simulink model "LAB7"  (R2025b)
settings: Solver=VariableStepAuto  StartTime=0.0  StopTime=100  RelTol=1e-3
settings Model: Creator=Wingshingsho  LastModifiedBy=Wingshingsho

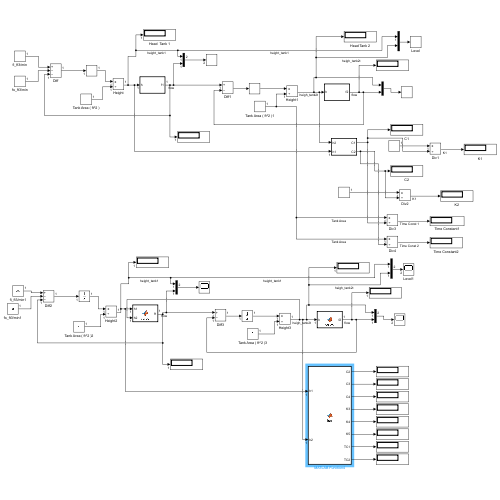
[thumbnail: Simulink's stored preview of the top-level diagram]
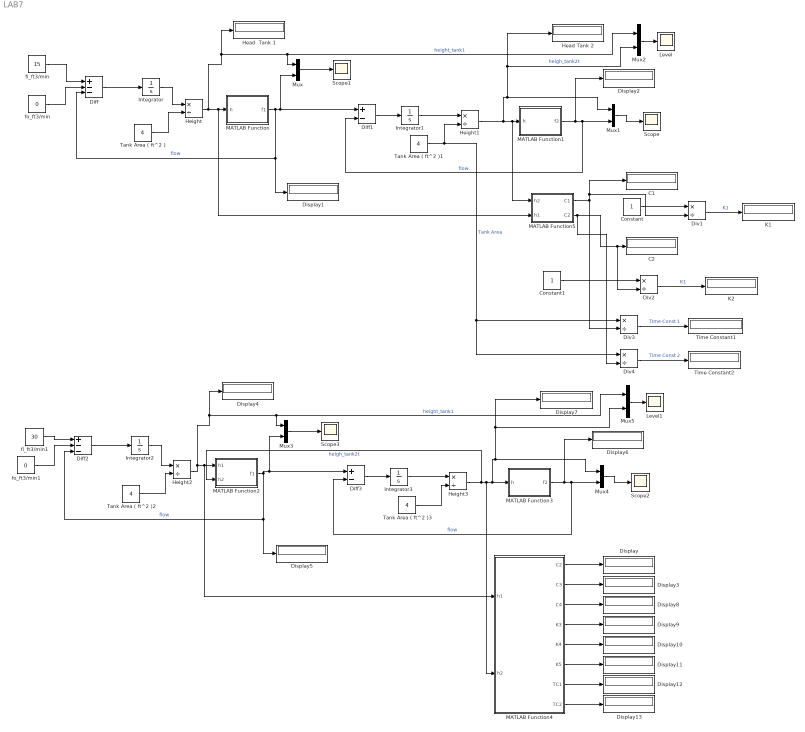
== system LAB7 ==
  C1 : Display
  C2 : Display
  Constant : Constant
  Constant1 : Constant
  Diff : Sum  Inputs=+--
  Diff1 : Sum  Inputs=+-
  Diff2 : Sum  Inputs=+--
  Diff3 : Sum  Inputs=+-
  Display{,1..13} (14 alike) : Display
  Div{1..4} (4 alike) : Product  Inputs=*/
  Head  Tank 1 : Display
  Head Tank 2 : Display
  Height{,1..3} (4 alike) : Product  Inputs=*/
  Integrator{,1..3} (4 alike) : Integrator
  K1 : Display
  K2 : Display
  Level : Scope
      settings: ActiveDisplayYMinimum=-1  ActiveDisplayYMaximum=1  DataLoggingVariableName=ScopeData2
  Level1 : Scope
      settings: ActiveDisplayYMinimum=-5.1866326305686812  ActiveDisplayYMaximum=46.679693675118138  DataLoggingVariableName=ScopeData3
  MATLAB Function : MATLAB Function  TreatAsAtomicUnit=on
  MATLAB Function1 : MATLAB Function  TreatAsAtomicUnit=on
  MATLAB Function2 : MATLAB Function  TreatAsAtomicUnit=on
  MATLAB Function3 : MATLAB Function  TreatAsAtomicUnit=on
  MATLAB Function4 : MATLAB Function  TreatAsAtomicUnit=on
  MATLAB Function5 : MATLAB Function  TreatAsAtomicUnit=on
  Mux{,1..5} (6 alike) : Mux  Inputs=2
  Scope{,1..3} (4 alike) : Scope
      Scope settings: ActiveDisplayYMinimum=-1  ActiveDisplayYMaximum=1
      Scope1 settings: ActiveDisplayYMinimum=-1  ActiveDisplayYMaximum=1
      Scope2 settings: ActiveDisplayYMinimum=-1  ActiveDisplayYMaximum=1  DataLoggingVariableName=ScopeData4
      Scope3 settings: ActiveDisplayYMinimum=-3.7438754161647805  ActiveDisplayYMaximum=33.694878745483031  DataLoggingVariableName=ScopeData5
  Tank Area ( ft^2 ){,1..3} (4 alike) : Constant  Value=4
  Time Constant1 : Display
  Time Constant2 : Display
  fi_ft3/min : Constant  Value=15
  fi_ft3/min1 : Constant  Value=30
  fo_ft3/min : Constant  Value=0
  fo_ft3/min1 : Constant  Value=0
  wires:
  fi_ft3/min/1 -> Diff/1
  fo_ft3/min/1 -> Diff/2
  Diff/1 -> Integrator/1
  Integrator/1 -> Height/1
  Tank Area ( ft^2 )/1 -> Height/2
  Height/1 -> Head  Tank 1/1, Mux2/1, Mux/1, MATLAB Function5/2(h1), MATLAB Function/1(h)  "height_tank1"
  MATLAB Function/1(f1) -> Diff/3, Display1/1, Diff1/1, Mux/2  "flow"
  Diff1/1 -> Integrator1/1
  Integrator1/1 -> Height1/1
  Tank Area ( ft^2 )1/1 -> Div4/1, Div3/1, Height1/2  "Tank Area"
  Height1/1 -> Mux2/2, Head Tank 2/1, Mux1/1, MATLAB Function5/1(h2), MATLAB Function1/1(h)  "heigh_tank2t"
  MATLAB Function1/1(f2) -> Display2/1, Mux1/2, Diff1/2  "flow"
  Mux/1 -> Scope1/1
  Mux1/1 -> Scope/1
  Mux2/1 -> Level/1
  Mux4/1 -> Scope2/1
  Height3/1 -> MATLAB Function2/2(h2), MATLAB Function4/2(h2), Mux5/2, Display7/1, Mux4/1, MATLAB Function3/1(h)  "heigh_tank2t"
  Mux3/1 -> Scope3/1
  MATLAB Function3/1(f2) -> Display6/1, Mux4/2, Diff3/2  "flow"
  Tank Area ( ft^2 )3/1 -> Height3/2
  Mux5/1 -> Level1/1
  MATLAB Function2/1(f1) -> Diff3/1, Mux3/2, Diff2/3, Display5/1  "flow"
  Height2/1 -> Display4/1, Mux5/1, Mux3/1, MATLAB Function4/1(h1), MATLAB Function2/1(h1)  "height_tank1"
  Integrator3/1 -> Height3/1
  Diff3/1 -> Integrator3/1
  Diff2/1 -> Integrator2/1
  fo_ft3/min1/1 -> Diff2/2
  fi_ft3/min1/1 -> Diff2/1
  Integrator2/1 -> Height2/1
  Tank Area ( ft^2 )2/1 -> Height2/2
  MATLAB Function5/1(C1) -> Div1/2, C1/1, Div3/2
  MATLAB Function5/2(C2) -> Div4/2, Div2/2, C2/1
  Constant/1 -> Div1/1
  Div1/1 -> K1/1  "K1"
  Constant1/1 -> Div2/1
  Div2/1 -> K2/1  "K1"
  Div3/1 -> Time Constant1/1  "TIme Const 1"
  Div4/1 -> Time Constant2/1  "Time Const 2"
  MATLAB Function4/1(C2) -> Display/1
  MATLAB Function4/2(C3) -> Display3/1
  MATLAB Function4/3(C4) -> Display8/1
  MATLAB Function4/4(K3) -> Display9/1
  MATLAB Function4/5(K4) -> Display10/1
  MATLAB Function4/6(K5) -> Display11/1
  MATLAB Function4/7(TC1) -> Display12/1
  MATLAB Function4/8(TC2) -> Display13/1

== matlab function LAB7/MATLAB Function1 ==
  data: h input; f2 output
function f2 = valve(h)
Cv = 75 * 0.13336;
LHO = 70;
SG = LHO / 62.4;
Pressure = ( LHO * h )/144;
f2 = Cv * (SG)^-0.5 * ((Pressure)^0.5);

end

== matlab function LAB7/MATLAB Function ==
  data: h input; f1 output
function f1 = valve(h)
Cv = 75 * 0.13336;
LHO = 70;
SG = LHO / 62.4;
Pressure = ( LHO * h )/144;
f1 = Cv * (SG)^-0.5 * ((Pressure)^0.5);

end

== matlab function LAB7/MATLAB Function2 ==
  data: h1 input; f1 output; h2 input
function f1 = valve(h1,h2)
Cv = 75 * 0.13336;
LHO = 70;
SG = LHO / 62.4;
Pressure = ( LHO * (h1-h2) )/144;
if Pressure > 0
    f1 = Cv * (SG)^-0.5 * ((Pressure)^0.5);
else
    f1 = 0;
end

end

== matlab function LAB7/MATLAB Function3 ==
  data: h input; f2 output
function f2 = valve(h)
Cv = 75 * 0.13336;
LHO = 70;
SG = LHO / 62.4;
Pressure = ( LHO * h )/144;
f2 = Cv * (SG)^-0.5 * ((Pressure)^0.5);

end

== matlab function LAB7/MATLAB Function4 ==
  data: h1 input; C2 output; h2 input; C3 output; C4 output; K3 output; K4 output; K5 output; TC1 output; TC2 output
function [C2,C3,C4,K3,K4,K5,TC1,TC2] = fcn(h1,h2)

CV = 75 * 0.134;
Density = 70;
SG = Density/62.4;
P1 = (Density * h1);
P2 = (Density * h2);
if h2 >= 0
    C3 = CV * 0.5 * sqrt(Density/(144*SG)) * ((h1-h2)^-0.5);
    C4 = CV * 0.5 * sqrt(Density/(144*SG)) * ((h1-h2)^-0.5) * (-1);
    C2 = CV * 0.5 * sqrt(Density/(144*SG)) * (h2^-0.5);
else
    C3 = 0;
    C4 = 0;
    C2 = 0;
end

K3 = 0;
K4 = 0;
K5 = 0;
TC1 = 0;
TC2 = 0;

== matlab function LAB7/MATLAB Function5 ==
  data: h2 input; C1 output; h1 input; C2 output
function [C1,C2] = linear(h2,h1)

Cv = 75 * 0.134;
Density = 70;
SG = Density / 62.4;
P1 = (Density * h1) / 144;
P2 = (Density * h2) / 144;
C1 = Cv * 0.5 * sqrt(Density/(144*SG)) * (h1^-0.5);
if h2 >= 0
    C2 = Cv * 0.5 * sqrt(Density/(144*SG)) * (h2^-0.5);
else
    C2 = 0;
end
